simulink model "openLoopR2019"  (R2021b)
settings: Solver=FixedStepAuto  StartTime=0.0  StopTime=inf  FixedStep=0.001  RelTol=1e-3
undefined symbols (not defined in the file or in its folder): a
settings Model: Creator=marko  LastModifiedBy=marko
settings SolverCC: AlgebraicLoopSolver=TrustRegion
settings DebuggingCC: SFMachineParentedDataDiag=warning

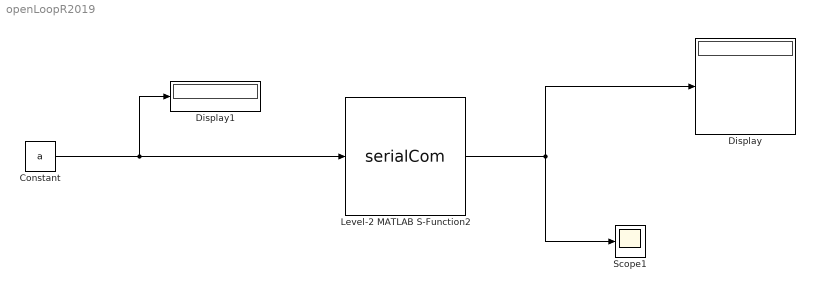
== system openLoopR2019 ==
  Constant : Constant  Value=a
  Display : Display
  Display1 : Display
  Level-2 MATLAB S-Function2 : M-S-Function  FunctionName=serialCom  Parameters='COM7', 115200
  Scope1 : Scope
  wires:
  Level-2 MATLAB S-Function2/1 -> Scope1/1, Display/1
  Constant/1 -> Display1/1, Level-2 MATLAB S-Function2/1
